simulink model "Plant"  (Simulink 7.5)
settings: Solver=ode15s  StartTime=0.0  StopTime=10.0  RelTol=1e-3
libraries: fl_lib x58, nesl_utility x6
settings Model: Creator=fguerin  LastModifiedBy=fguerin
settings DataIOCC: LimitDataPoints=off  SaveFormat=Structure  SaveOutput=off  SignalLogging=off  SaveTime=off
settings OptimizationCC: InlineParams=on  InlineInvariantSignals=on  EnhancedBackFolding=on  StrengthReduction=on  EnforceIntegerDowncast=off  OptimizeModelRefInitCode=on  LifeSpan=Inf
settings DebuggingCC: StrictBusMsg=Warning
settings HardwareCC: ProdIntDivRoundTo=Zero  ProdEndianess=LittleEndian  ProdHWDeviceType=Freescale->MPC5500
settings RTWCC: SystemTargetFile=ert.tlc  TemplateMakefile=ert_default_tmf  Description=Real-Time Workshop Embedded Coder  GenerateReport=on  ProcessScript=ert_make_rtw_hook  IncludeHyperlinkInReport=on  LaunchReport=on  GenerateTraceInfo=on  GenerateTraceReport=on  GenerateTraceReportSl=on  GenerateTraceReportSf=on  GenerateTraceReportEml=on
settings CodeAppCC: IgnoreCustomStorageClasses=off
settings ERTTargetCC: UtilityFuncGeneration=Shared location  MultiwordLength=2048  GenerateSampleERTMain=on  IncludeMdlTerminateFcn=off  SuppressErrorStatus=on  ERTCustomFileTemplate=example_file_process.tlc  ConvertIfToSwitch=off

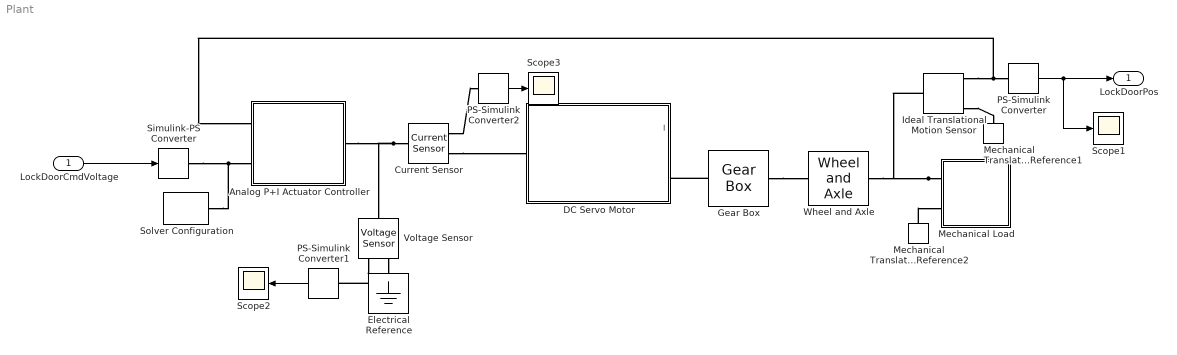
== system Plant ==
  LockDoorCmdVoltage : Inport  PortDimensions=1  SampleTime=[0,1]  DataType=double  OutDataType=fixdt(1, 16)  OutScaling=2^0  OutDataTypeStr=double
  Analog P+I Actuator Controller : Subsystem  mask{prox_sens=1}
      mask prompts: prox_sens "Proximity Sensitivity (V/mm)"
      mask Display:
      | image(imread('Analog_PI_Controller.jpg'))
      | color('red')
      | port_label('lconn',1,'y')
      | port_label('lconn',2,'R')
      | port_label('rconn',1,'Vi')
  Current Sensor : fl_lib/Electrical/Electrical Sensors/Current Sensor  DialogController=NetworkEngine.DynNeDlgSource  SystemSampleTime=-1  i1_Log=off  v1_Log=off  LocalVarNames=|i1|v1  LocalVarDescs=|i1|v1  LocalVarLogging=[0 0]
  DC Servo Motor : Subsystem  mask{G=1e-4/(pi/2), J=1e-6, lambda=0.07, R=10, L=2.5, Kt=0.04, x_max=0.5}
      mask prompts: G "Spool displacement per motor rotation"; J "Total inertia reflected to motor (kg m^2)"; lambda "Total damping reflected to motor (Nm/(rad/s))"; R "Torque motor winding resistance (ohms)"; L "Torque motor winding inductance (H)"; Kt "Torque motor torque constant (Nm/A)"; x_max "Spool displacement limit (mm)"
      mask Display:
      | image(imread('DC_Motor_Image.jpg'))
      | color('red')
      | port_label('lconn',1,'Vi')
      | port_label('rconn',1,'R')
      | port_label('output',1,'I')
  Electrical Reference : fl_lib/Electrical/Electrical Elements/Electrical Reference  DialogController=NetworkEngine.DynNeDlgSource  SystemSampleTime=-1  i_Log=off  LocalVarNames=|i  LocalVarDescs=|i  LocalVarLogging=0
  Gear Box : fl_lib/Mechanical/Mechanisms/Gear Box  DialogController=NetworkEngine.DynNeDlgSource  SystemSampleTime=-1  ratio=2  t_in_Log=off  t_out_Log=off  LocalVarNames=|t_in|t_out  LocalVarDescs=|t_in|t_out  LocalVarLogging=[0 0]
  Ideal Translational Motion Sensor : fl_lib/Mechanical/Mechanical Sensors/Ideal Translational Motion Sensor  DialogController=NetworkEngine.DynNeDlgSource  SystemSampleTime=-1  offset=0 m  v_Log=off  f_Log=off  x_Log=off  LocalVarNames=|v|f|x  LocalVarDescs=|v|f|x  LocalVarLogging=[0 0 0]
  Mechanical Load : Subsystem  mask{m=0.05, k=1e-6, c=1e-6, stroke=100}
      mask prompts: m "Mass (kg)"; k "Spring Stiffness (N/mm)"; c "Damping Coefficient (N/(mm/s))"; stroke "Stroke Distance (mm)"
      mask Display:
      | image(imread('Spring_Damper_Load.jpg'))
      | color('red')
      | port_label('lconn',1,'R')
      | port_label('lconn',2,'C')
  Mechanical Translational Reference1 : fl_lib/Mechanical/Translational Elements/Mechanical Translational Reference  DialogController=NetworkEngine.DynNeDlgSource  SystemSampleTime=-1  f_Log=off  LocalVarNames=|f  LocalVarDescs=|f  LocalVarLogging=0
  Mechanical Translational Reference2 : fl_lib/Mechanical/Translational Elements/Mechanical Translational Reference  DialogController=NetworkEngine.DynNeDlgSource  SystemSampleTime=-1  f_Log=off  LocalVarNames=|f  LocalVarDescs=|f  LocalVarLogging=0
  PS-Simulink Converter : nesl_utility/PS-Simulink Converter  DialogController=NetworkEngine.DynNeUtilDlgSource  SystemSampleTime=-1  PhysicalDomain=network_engine_domain  LeftPortType=input  RightPortType=output  SubClassName=ps_output  Unit=mm  AffineConversion=off
  PS-Simulink Converter1 : nesl_utility/PS-Simulink Converter  DialogController=NetworkEngine.DynNeUtilDlgSource  SystemSampleTime=-1  PhysicalDomain=network_engine_domain  LeftPortType=input  RightPortType=output  SubClassName=ps_output  Unit=V  AffineConversion=off
  PS-Simulink Converter2 : nesl_utility/PS-Simulink Converter  DialogController=NetworkEngine.DynNeUtilDlgSource  SystemSampleTime=-1  PhysicalDomain=network_engine_domain  LeftPortType=input  RightPortType=output  SubClassName=ps_output  Unit=mA  AffineConversion=off
  Scope1 : Scope
      settings: TimeRange=10  SaveName=ScopeData2
  Scope2 : Scope
  Scope3 : Scope
      settings: TimeRange=10
  Simulink-PS Converter : nesl_utility/Simulink-PS Converter  DialogController=NetworkEngine.DynNeUtilDlgSource  SystemSampleTime=-1  PhysicalDomain=network_engine_domain  LeftPortType=input  RightPortType=output  SubClassName=ps_input  Unit=V  AffineConversion=off  InputFilterTimeConstant=.001  UdotUserProvided=0
  Solver Configuration : nesl_utility/Solver Configuration  DialogController=NetworkEngine.DynNeUtilDlgSource  SystemSampleTime=-1  PhysicalDomain=network_engine_domain  LeftPortType=input  RightPortType=generic  SubClassName=solver  Accelerate=off  Profile=off  ResidualTolerance=1e-9  MaxNonlinIter=3  MaxModeIter=2  DoFixedCost=off  UseLocalSampling=off  DoDC=off  LinearAlgebra=Sparse  LocalSolverSampleTime=.001  LocalSolverChoice=NE_BACKWARD_EULER_ADVANCER  UseLocalSolver=off
  Voltage Sensor : fl_lib/Electrical/Electrical Sensors/Voltage Sensor  DialogController=NetworkEngine.DynNeDlgSource  SystemSampleTime=-1  i1_Log=off  v1_Log=off  LocalVarNames=|i1|v1  LocalVarDescs=|i1|v1  LocalVarLogging=[0 0]
  Wheel and Axle : fl_lib/Mechanical/Mechanisms/Wheel and Axle  DialogController=NetworkEngine.DynNeDlgSource  SystemSampleTime=-1  R=0.05 m  or=1  torque_A_Log=off  force_P_Log=off  ang_velocity_Log=off  velocity_Log=off  LocalVarNames=|torque_A|force_P|ang_velocity|velocity  LocalVarDescs=|Axle torque (N*m)|Periphery force (N)|Axle angular velocity (rad/s)|Periphery velocity (m/s)  LocalVarLogging=[0 0 0 0]
  LockDoorPos : Outport  PortDimensions=1  SampleTime=0  DataType=double  OutDataType=fixdt(1, 16)  OutScaling=2^0  OutDataTypeStr=double
  wires:
  PS-Simulink Converter2/1 -> Scope3/1
  PS-Simulink Converter1/1 -> Scope2/1
  PS-Simulink Converter/1 -> Scope1/1, LockDoorPos/1
  LockDoorCmdVoltage/1 -> Simulink-PS Converter/1
  connections:
  Mechanical Translational Reference2/LConn1 -- Mechanical Load/LConn2
  Voltage Sensor/RConn1 -- PS-Simulink Converter1/LConn1
  Gear Box/RConn1 -- Wheel and Axle/LConn1
  Voltage Sensor/RConn2 -- Electrical Reference/LConn1
  Ideal Translational Motion Sensor/RConn1 -- Mechanical Translational Reference1/LConn1
  Current Sensor/RConn2 -- DC Servo Motor/LConn1
  Gear Box/LConn1 -- DC Servo Motor/RConn1
  Solver Configuration/RConn1 -- Analog P+I Actuator Controller/LConn2 -- Simulink-PS Converter/RConn1
  Current Sensor/RConn1 -- PS-Simulink Converter2/LConn1
  PS-Simulink Converter/LConn1 -- Ideal Translational Motion Sensor/RConn3 -- Analog P+I Actuator Controller/LConn1
  Mechanical Load/LConn1 -- Ideal Translational Motion Sensor/LConn1 -- Wheel and Axle/RConn1
  Analog P+I Actuator Controller/RConn1 -- Voltage Sensor/LConn1 -- Current Sensor/LConn1

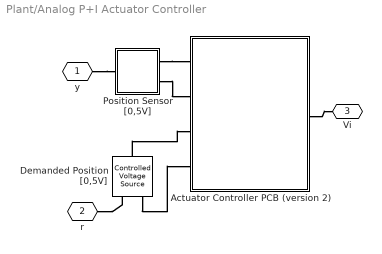
== system Plant/Analog P+I Actuator Controller ==
  Actuator Controller PCB (version 2) : Subsystem
      mask Display:
      | image(imread('pcb.jpg'))
      | color('red')
      | port_label('lconn',1,'P+')
      | port_label('lconn',2,'P-')
      | port_label('lconn',3,'D+')
      | port_label('lconn',4,'D-')
      | port_label('rconn',1,'Vi')
  Demanded Position [0,5V] : fl_lib/Electrical/Electrical Sources/Controlled Voltage Source  DialogController=NetworkEngine.DynNeDlgSource  SystemSampleTime=-1  i_Log=off  v_Log=off  LocalVarNames=|current|voltage|power  LocalVarDescs=|Current (A)|Voltage (V)|Power (W)  LocalVarLogging=[0 0 0]
  Position Sensor [0,5V] : Subsystem
  y : PMIOPort  Tag=PMCPort  Port=1  Side=Left
  r : PMIOPort  Tag=PMCPort  Port=2  Side=Left
  Vi : PMIOPort  Port=3  Side=Right
  connections:
  r/RConn1 -- Demanded Position [0,5V]/RConn1
  y/RConn1 -- Position Sensor [0,5V]/LConn1
  Actuator Controller PCB (version 2)/RConn1 -- Vi/RConn1
  Position Sensor [0,5V]/RConn1 -- Actuator Controller PCB (version 2)/LConn1
  Position Sensor [0,5V]/RConn2 -- Actuator Controller PCB (version 2)/LConn2
  Demanded Position [0,5V]/LConn1 -- Actuator Controller PCB (version 2)/LConn3
  Demanded Position [0,5V]/RConn2 -- Actuator Controller PCB (version 2)/LConn4

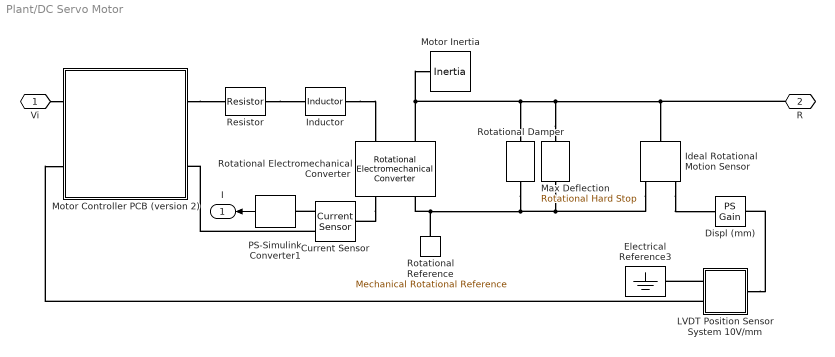
== system Plant/DC Servo Motor ==
  Current Sensor : fl_lib/Electrical/Electrical Sensors/Current Sensor  DialogController=NetworkEngine.DynNeDlgSource  SystemSampleTime=-1  i1_Log=off  v1_Log=off  LocalVarNames=|i1|v1  LocalVarDescs=|i1|v1  LocalVarLogging=[]
  Displ (mm) : fl_lib/Physical Signals/Functions/PS Gain  DialogController=NetworkEngine.DynNeDlgSource  SystemSampleTime=-1  gain=G*1000  LocalVarLogging=[]
  Electrical Reference3 : fl_lib/Electrical/Electrical Elements/Electrical Reference  DialogController=NetworkEngine.DynNeDlgSource  SystemSampleTime=-1  i_Log=off  LocalVarNames=|i  LocalVarDescs=|i  LocalVarLogging=[]
  Ideal Rotational Motion Sensor : fl_lib/Mechanical/Mechanical Sensors/Ideal Rotational Motion Sensor  DialogController=NetworkEngine.DynNeDlgSource  SystemSampleTime=-1  offset=0 deg  w_Log=off  t_Log=off  phi_Log=off  LocalVarNames=|w|t|phi  LocalVarDescs=|w|t|phi  LocalVarLogging=[]
  Inductor : fl_lib/Electrical/Electrical Elements/Inductor  DialogController=NetworkEngine.DynNeDlgSource  SystemSampleTime=-1  l=L H  i0=0 A  r=0 Ohm  g=1e-09 1/Ohm  i_Log=off  v_Log=off  i_L_Log=off  LocalVarNames=|current|voltage|power  LocalVarDescs=|Inductor current (A) |Voltage across inductor (V)|Power (W)  LocalVarLogging=[0 0 0]
  LVDT Position Sensor System 10V/mm : Subsystem
  Max Deflection : fl_lib/Mechanical/Rotational Elements/Rotational Hard Stop  DialogController=NetworkEngine.DynNeDlgSource  SystemSampleTime=-1  upper_bnd=x_max*1e-3/G rad  lower_bnd=-x_max*1e-3/G rad  stiff_up=1e+06 N*m/rad  stiff_low=1e+06 N*m/rad  D_up=0.05 N*m/(rad/s)  D_low=0.05 N*m/(rad/s)  t_Log=off  w_Log=off  phi_Log=off  LocalVarNames=|contact_torque|rel_angle  LocalVarDescs=|Contact torque (N*m)|Slider-case relative angle (rad)  LocalVarLogging=[0 0]
  Motor Controller PCB (version 2) : Subsystem
      mask Display:
      | image(imread('pcb.jpg'))
      | color('red')
      | port_label('lconn',1,'Vref')
      | port_label('lconn',2,'Vm')
      | port_label('rconn',1,'M+')
      | port_label('rconn',2,'M-')
  Motor Inertia : fl_lib/Mechanical/Rotational Elements/Inertia  DialogController=NetworkEngine.DynNeDlgSource  SystemSampleTime=-1  inertia=J kg*m^2  initial_velocity=0 rad/s  t_Log=off  LocalVarNames=|torque|velocity  LocalVarDescs=|Inertia torque (N*m)|Inertia absolute velocity (rad/s)  LocalVarLogging=[0 0]
  PS-Simulink Converter1 : nesl_utility/PS-Simulink Converter  DialogController=NetworkEngine.DynNeUtilDlgSource  SystemSampleTime=-1  PhysicalDomain=network_engine_domain  LeftPortType=input  RightPortType=output  SubClassName=ps_output  Unit=1  AffineConversion=off
  Resistor : fl_lib/Electrical/Electrical Elements/Resistor  DialogController=NetworkEngine.DynNeDlgSource  SystemSampleTime=-1  R=R Ohm  i_Log=off  v_Log=off  LocalVarNames=|current|voltage|power  LocalVarDescs=|Resistor current (A)|Voltage across resistor (V)|Power (W)  LocalVarLogging=[0 0 0]
  Rotational Damper : fl_lib/Mechanical/Rotational Elements/Rotational Damper  DialogController=NetworkEngine.DynNeDlgSource  SystemSampleTime=-1  D=lambda N*m/(rad/s)  t_Log=off  w_Log=off  LocalVarNames=|torque|velocity|power  LocalVarDescs=|Damping torque (N*m)|Damper relative velocity (rad/s)|Power dissipated in the damper (W)  LocalVarLogging=[0 0 0]
  Rotational Electromechanical Converter : fl_lib/Electrical/Electrical Elements/Rotational Electromechanical Converter  DialogController=NetworkEngine.DynNeDlgSource  SystemSampleTime=-1  K=Kt V/(rad/s)  i_Log=off  v_Log=off  t_Log=off  w_Log=off  LocalVarNames=|current|voltage|power|torque|speed  LocalVarDescs=|Current (A)|Voltage (V)|Power (W)|Torque (Nm)|Angular speed (rad/s)  LocalVarLogging=[0 0 0 0 0]
  Rotational Reference : fl_lib/Mechanical/Rotational Elements/Mechanical Rotational Reference  DialogController=NetworkEngine.DynNeDlgSource  SystemSampleTime=-1  t_Log=off  LocalVarNames=|t  LocalVarDescs=|t  LocalVarLogging=[]
  Vi : PMIOPort  Port=1  Side=Left
  R : PMIOPort  Port=2  Side=Right
  I : Outport  OutDataType=sfix(16)  OutScaling=2^0
  wires:
  PS-Simulink Converter1/1 -> I/1
  connections:
  Ideal Rotational Motion Sensor/RConn3 -- Displ (mm)/LConn1
  LVDT Position Sensor System 10V/mm/RConn1 -- Electrical Reference3/LConn1
  Inductor/RConn1 -- Rotational Electromechanical Converter/LConn1
  Resistor/RConn1 -- Inductor/LConn1
  Current Sensor/RConn2 -- Motor Controller PCB (version 2)/RConn2
  LVDT Position Sensor System 10V/mm/RConn2 -- Motor Controller PCB (version 2)/LConn2
  Motor Controller PCB (version 2)/RConn1 -- Resistor/LConn1
  Rotational Electromechanical Converter/RConn1 -- Current Sensor/LConn1
  Current Sensor/RConn1 -- PS-Simulink Converter1/LConn1
  LVDT Position Sensor System 10V/mm/LConn1 -- Displ (mm)/RConn1
  Rotational Damper/RConn1 -- Rotational Electromechanical Converter/RConn2 -- Rotational Reference/LConn1 -- Ideal Rotational Motion Sensor/RConn1 -- Max Deflection/RConn1
  Max Deflection/LConn1 -- R/RConn1 -- Ideal Rotational Motion Sensor/LConn1 -- Motor Inertia/LConn1 -- Rotational Electromechanical Converter/LConn2 -- Rotational Damper/LConn1
  Vi/RConn1 -- Motor Controller PCB (version 2)/LConn1

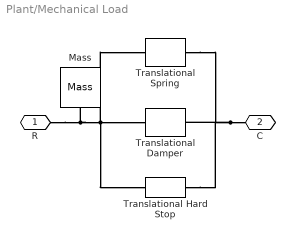
== system Plant/Mechanical Load ==
  Mass : fl_lib/Mechanical/Translational Elements/Mass  DialogController=NetworkEngine.DynNeDlgSource  SystemSampleTime=-1  mass=m kg  initial_velocity=0 m/s  f_Log=off  LocalVarNames=|force|velocity  LocalVarDescs=|Inertia force (N)|Mass absolute velocity (m/s)  LocalVarLogging=[0 0]
  Translational Damper : fl_lib/Mechanical/Translational Elements/Translational Damper  DialogController=NetworkEngine.DynNeDlgSource  SystemSampleTime=-1  D=c N/(mm/s)  f_Log=off  v_Log=off  LocalVarNames=|force|rel_velocity|power  LocalVarDescs=|Damping force (N)|Damper relative velocity (m/s)|Power dissipated in the damper (W)  LocalVarLogging=[0 0 0]
  Translational Hard Stop : fl_lib/Mechanical/Translational Elements/Translational Hard Stop  DialogController=NetworkEngine.DynNeDlgSource  SystemSampleTime=-1  upper_bnd=stroke/2 mm  lower_bnd=-stroke/2 mm  stiff_up=1e+07 N/m  stiff_low=1e+07 N/m  D_up=3000 N/(m/s)  D_low=3000 N/(m/s)  f_Log=off  v_Log=off  x_Log=off  LocalVarNames=|contact_force|rel_displacement  LocalVarDescs=|Contact force (N)|Slider-case relative displacement (m)  LocalVarLogging=[0 0]
  Translational Spring : fl_lib/Mechanical/Translational Elements/Translational Spring  DialogController=NetworkEngine.DynNeDlgSource  SystemSampleTime=-1  spr_rate=k N/mm  init_def=0 mm  f_Log=off  v_Log=off  x_Log=off  LocalVarNames=|force|deformation  LocalVarDescs=|Spring force (N)|Spring deformation (m)  LocalVarLogging=[0 0]
  R : PMIOPort  Port=1  Side=Left
  C : PMIOPort  Port=2  Side=Left
  connections:
  C/RConn1 -- Translational Hard Stop/RConn1 -- Translational Damper/RConn1 -- Translational Spring/RConn1
  Mass/LConn1 -- Translational Hard Stop/LConn1 -- Translational Damper/LConn1 -- Translational Spring/LConn1 -- R/RConn1

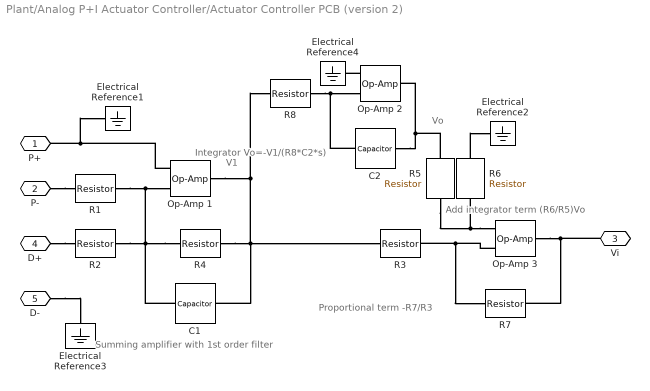
== system Plant/Analog P+I Actuator Controller/Actuator Controller PCB (version 2) ==
  note: V1
  note: Vo
  note: Add integrator
      | term (R6/R5)Vo
  note: Proportional
      | term -R7/R3
  note: Integrator
      | Vo=-V1/(R8*C2*s)
  note: Summing amplifier
      | with 1st order filter
  C1 : fl_lib/Electrical/Electrical Elements/Capacitor  DialogController=NetworkEngine.DynNeDlgSource  SystemSampleTime=-1  c=0.15e-6 F  v0=0 V  r=1e-06 Ohm  g=0 1/Ohm  i_Log=off  v_Log=off  vc_Log=off  LocalVarNames=|current|voltage|power  LocalVarDescs=|Capacitor current (A)|Voltage across capacitor (V)|Power (W)  LocalVarLogging=[0 0 0]
  C2 : fl_lib/Electrical/Electrical Elements/Capacitor  DialogController=NetworkEngine.DynNeDlgSource  SystemSampleTime=-1  c=100e-6 F  v0=0 V  r=1e-06 Ohm  g=0 1/Ohm  i_Log=off  v_Log=off  vc_Log=off  LocalVarNames=|current|voltage|power  LocalVarDescs=|Capacitor current (A)|Voltage across capacitor (V)|Power (W)  LocalVarLogging=[0 0 0]
  Electrical Reference{1..4} (4 alike) : fl_lib/Electrical/Electrical Elements/Electrical Reference  DialogController=NetworkEngine.DynNeDlgSource  SystemSampleTime=-1  i_Log=off  LocalVarNames=|i  LocalVarDescs=|i  LocalVarLogging=[]
  Op-Amp 1 : fl_lib/Electrical/Electrical Elements/Op-Amp  DialogController=NetworkEngine.DynNeDlgSource  SystemSampleTime=-1  i1_Log=off  v1_Log=off  outI_Log=off  LocalVarNames=|i1|v1|outI  LocalVarDescs=|i1|v1|outI  LocalVarLogging=[]
  Op-Amp 2 : fl_lib/Electrical/Electrical Elements/Op-Amp  DialogController=NetworkEngine.DynNeDlgSource  SystemSampleTime=-1  i1_Log=off  v1_Log=off  outI_Log=off  LocalVarNames=|i1|v1|outI  LocalVarDescs=|i1|v1|outI  LocalVarLogging=[]
  Op-Amp 3 : fl_lib/Electrical/Electrical Elements/Op-Amp  DialogController=NetworkEngine.DynNeDlgSource  SystemSampleTime=-1  i1_Log=off  v1_Log=off  outI_Log=off  LocalVarNames=|i1|v1|outI  LocalVarDescs=|i1|v1|outI  LocalVarLogging=[]
  R{1..3,5..6,8} (6 alike) : fl_lib/Electrical/Electrical Elements/Resistor  DialogController=NetworkEngine.DynNeDlgSource  SystemSampleTime=-1  R=10e3 Ohm  i_Log=off  v_Log=off  LocalVarNames=|current|voltage|power  LocalVarDescs=|Resistor current (A)|Voltage across resistor (V)|Power (W)  LocalVarLogging=[0 0 0]
  R4 : fl_lib/Electrical/Electrical Elements/Resistor  DialogController=NetworkEngine.DynNeDlgSource  SystemSampleTime=-1  R=5.7e3 Ohm  i_Log=off  v_Log=off  LocalVarNames=|current|voltage|power  LocalVarDescs=|Resistor current (A)|Voltage across resistor (V)|Power (W)  LocalVarLogging=[0 0 0]
  R7 : fl_lib/Electrical/Electrical Elements/Resistor  DialogController=NetworkEngine.DynNeDlgSource  SystemSampleTime=-1  R=20e3 Ohm  i_Log=off  v_Log=off  LocalVarNames=|current|voltage|power  LocalVarDescs=|Resistor current (A)|Voltage across resistor (V)|Power (W)  LocalVarLogging=[0 0 0]
  P+ : PMIOPort  Port=1  Side=Left
  P- : PMIOPort  Port=2  Side=Left
  Vi : PMIOPort  Port=3  Side=Right
  D+ : PMIOPort  Port=4  Side=Left
  D- : PMIOPort  Port=5  Side=Left
  connections:
  D+/RConn1 -- R2/LConn1
  Op-Amp 2/LConn1 -- Electrical Reference4/LConn1
  D-/RConn1 -- Electrical Reference3/LConn1
  R6/RConn1 -- Electrical Reference2/LConn1
  P-/RConn1 -- R1/LConn1
  Op-Amp 3/LConn2 -- R7/LConn1 -- R3/RConn1
  Op-Amp 3/LConn1 -- R6/LConn1 -- R5/RConn1
  Op-Amp 3/RConn1 -- Vi/RConn1 -- R7/RConn1
  Op-Amp 1/LConn1 -- Electrical Reference1/LConn1 -- P+/RConn1
  C2/RConn1 -- Op-Amp 2/RConn1 -- R5/LConn1
  C2/LConn1 -- R8/RConn1 -- Op-Amp 2/LConn2
  R4/RConn1 -- C1/RConn1 -- Op-Amp 1/RConn1 -- R8/LConn1 -- R3/LConn1
  R4/LConn1 -- R2/RConn1 -- Op-Amp 1/LConn2 -- R1/RConn1 -- C1/LConn1

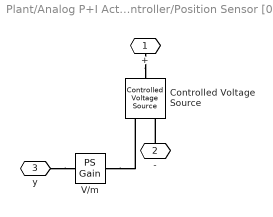
== system Plant/Analog P+I Actuator Controller/Position Sensor [0,5V] ==
  Controlled Voltage Source : fl_lib/Electrical/Electrical Sources/Controlled Voltage Source  DialogController=NetworkEngine.DynNeDlgSource  SystemSampleTime=-1  i_Log=off  v_Log=off  LocalVarNames=|current|voltage|power  LocalVarDescs=|Current (A)|Voltage (V)|Power (W)  LocalVarLogging=[0 0 0]
  V/m : fl_lib/Physical Signals/Functions/PS Gain  DialogController=NetworkEngine.DynNeDlgSource  SystemSampleTime=-1  gain=prox_sens*1000  LocalVarLogging=[]
  + : PMIOPort  Port=1  Side=Right
  - : PMIOPort  Port=2  Side=Right
  y : PMIOPort  Port=3  Side=Left
  connections:
  y/RConn1 -- V/m/LConn1
  -/RConn1 -- Controlled Voltage Source/RConn2
  +/RConn1 -- Controlled Voltage Source/LConn1
  V/m/RConn1 -- Controlled Voltage Source/RConn1

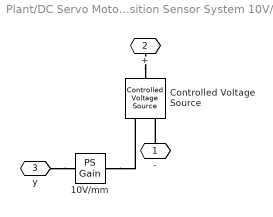
== system Plant/DC Servo Motor/LVDT Position Sensor System 10V/mm ==
  10V/mm : fl_lib/Physical Signals/Functions/PS Gain  DialogController=NetworkEngine.DynNeDlgSource  SystemSampleTime=-1  gain=10  LocalVarLogging=[]
  Controlled Voltage Source : fl_lib/Electrical/Electrical Sources/Controlled Voltage Source  DialogController=NetworkEngine.DynNeDlgSource  SystemSampleTime=-1  i_Log=off  v_Log=off  LocalVarNames=|current|voltage|power  LocalVarDescs=|Current (A)|Voltage (V)|Power (W)  LocalVarLogging=[0 0 0]
  - : PMIOPort  Port=1  Side=Right
  + : PMIOPort  Port=2  Side=Right
  y : PMIOPort  Port=3  Side=Left
  connections:
  y/RConn1 -- 10V/mm/LConn1
  -/RConn1 -- Controlled Voltage Source/RConn2
  +/RConn1 -- Controlled Voltage Source/LConn1
  10V/mm/RConn1 -- Controlled Voltage Source/RConn1

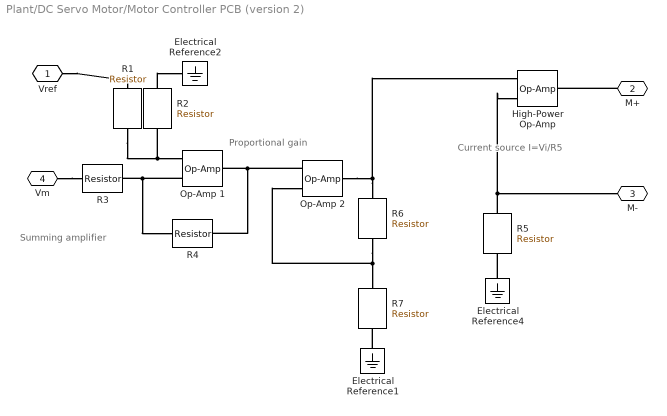
== system Plant/DC Servo Motor/Motor Controller PCB (version 2) ==
  note: Current source
      | I=Vi/R5
  note: Summing
      | amplifier
  note: Proportional gain
  Electrical Reference1 : fl_lib/Electrical/Electrical Elements/Electrical Reference  DialogController=NetworkEngine.DynNeDlgSource  SystemSampleTime=-1  i_Log=off  LocalVarNames=|i  LocalVarDescs=|i  LocalVarLogging=[]
  Electrical Reference2 : fl_lib/Electrical/Electrical Elements/Electrical Reference  DialogController=NetworkEngine.DynNeDlgSource  SystemSampleTime=-1  i_Log=off  LocalVarNames=|i  LocalVarDescs=|i  LocalVarLogging=[]
  Electrical Reference4 : fl_lib/Electrical/Electrical Elements/Electrical Reference  DialogController=NetworkEngine.DynNeDlgSource  SystemSampleTime=-1  i_Log=off  LocalVarNames=|i  LocalVarDescs=|i  LocalVarLogging=[]
  High-Power Op-Amp : fl_lib/Electrical/Electrical Elements/Op-Amp  DialogController=NetworkEngine.DynNeDlgSource  SystemSampleTime=-1  i1_Log=off  v1_Log=off  outI_Log=off  LocalVarNames=|i1|v1|outI  LocalVarDescs=|i1|v1|outI  LocalVarLogging=[]
  Op-Amp 1 : fl_lib/Electrical/Electrical Elements/Op-Amp  DialogController=NetworkEngine.DynNeDlgSource  SystemSampleTime=-1  i1_Log=off  v1_Log=off  outI_Log=off  LocalVarNames=|i1|v1|outI  LocalVarDescs=|i1|v1|outI  LocalVarLogging=[]
  Op-Amp 2 : fl_lib/Electrical/Electrical Elements/Op-Amp  DialogController=NetworkEngine.DynNeDlgSource  SystemSampleTime=-1  i1_Log=off  v1_Log=off  outI_Log=off  LocalVarNames=|i1|v1|outI  LocalVarDescs=|i1|v1|outI  LocalVarLogging=[]
  R{1..3,7} (4 alike) : fl_lib/Electrical/Electrical Elements/Resistor  DialogController=NetworkEngine.DynNeDlgSource  SystemSampleTime=-1  R=10e3 Ohm  i_Log=off  v_Log=off  LocalVarNames=|current|voltage|power  LocalVarDescs=|Resistor current (A)|Voltage across resistor (V)|Power (W)  LocalVarLogging=[0 0 0]
  R4 : fl_lib/Electrical/Electrical Elements/Resistor  DialogController=NetworkEngine.DynNeDlgSource  SystemSampleTime=-1  R=100e3 Ohm  i_Log=off  v_Log=off  LocalVarNames=|current|voltage|power  LocalVarDescs=|Resistor current (A)|Voltage across resistor (V)|Power (W)  LocalVarLogging=[0 0 0]
  R5 : fl_lib/Electrical/Electrical Elements/Resistor  DialogController=NetworkEngine.DynNeDlgSource  SystemSampleTime=-1  R=50 Ohm  i_Log=off  v_Log=off  LocalVarNames=|current|voltage|power  LocalVarDescs=|Resistor current (A)|Voltage across resistor (V)|Power (W)  LocalVarLogging=[0 0 0]
  R6 : fl_lib/Electrical/Electrical Elements/Resistor  DialogController=NetworkEngine.DynNeDlgSource  SystemSampleTime=-1  R=100e3 Ohm  i_Log=off  v_Log=off  LocalVarNames=|current|voltage|power  LocalVarDescs=|Resistor current (A)|Voltage across resistor (V)|Power (W)  LocalVarLogging=[0 0 0]
  Vref : PMIOPort  Port=1  Side=Left
  M+ : PMIOPort  Port=2  Side=Right
  M- : PMIOPort  Port=3  Side=Right
  Vm : PMIOPort  Port=4  Side=Left
  connections:
  R6/LConn1 -- Op-Amp 2/RConn1 -- High-Power Op-Amp/LConn1
  R5/LConn1 -- High-Power Op-Amp/LConn2 -- M-/RConn1
  R1/RConn1 -- R2/LConn1 -- Op-Amp 1/LConn1
  R3/RConn1 -- R4/LConn1 -- Op-Amp 1/LConn2
  R4/RConn1 -- Op-Amp 2/LConn1 -- Op-Amp 1/RConn1
  R6/RConn1 -- Op-Amp 2/LConn2 -- R7/LConn1
  M+/RConn1 -- High-Power Op-Amp/RConn1
  Electrical Reference1/LConn1 -- R7/RConn1
  Electrical Reference4/LConn1 -- R5/RConn1
  Vm/RConn1 -- R3/LConn1
  Vref/RConn1 -- R1/LConn1
  R2/RConn1 -- Electrical Reference2/LConn1
